simulink model "impulse_ex_3"  (R2024a)
settings: Solver=VariableStepAuto  StartTime=0.0  StopTime=10  RelTol=1e-6  AbsTol=1e-6
values from neighbouring files (symbols this model uses):
  a = 0.001    [impulseDD.sldd]
undefined symbols (not defined in the file or in its folder): sys
libraries: simulink x1
settings Model: DataDictionary=impulseDD.sldd  Creator=grouleau  LastModifiedBy=grouleau

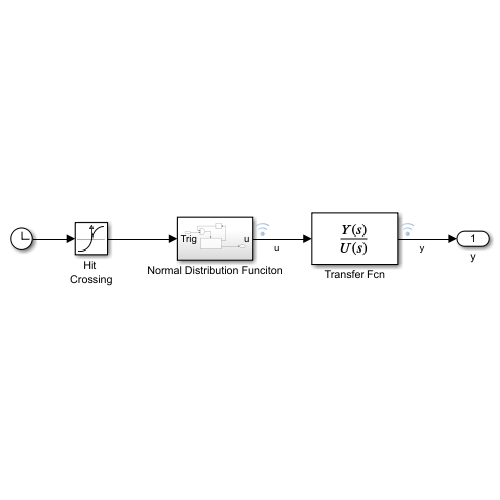
[thumbnail: Simulink's stored preview of the top-level diagram]
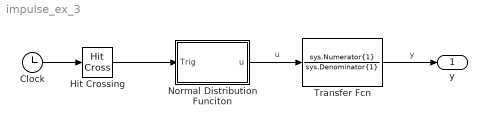
== system impulse_ex_3 ==
  Clock : Clock
  Hit Crossing : HitCross  HitCrossingOffset=1.23456  HitCrossingDirection=rising
  Normal Distribution Funciton : Subsystem
  Transfer Fcn : TransferFcn  Numerator=sys.Numerator{1}  Denominator=sys.Denominator{1}
  y : Outport
  wires:
  Transfer Fcn/1 -> y/1  "y"
  Clock/1 -> Hit Crossing/1
  Normal Distribution Funciton/1(u) -> Transfer Fcn/1  "u"
  Hit Crossing/1 -> Normal Distribution Funciton/1(Trig)

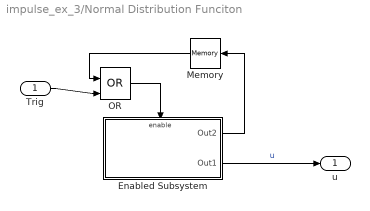
== system impulse_ex_3/Normal Distribution Funciton ==
  Trig : Inport
  Enabled Subsystem : Subsystem  TreatAsAtomicUnit=on
  Memory : Memory
  OR : Logic  Operator=OR  IconShape=distinctive  AllPortsSameDT=off  OutDataTypeStr=boolean
  u : Outport
  wires:
  Enabled Subsystem/2(Out1) -> u/1  "u"
  Enabled Subsystem/1(Out2) -> Memory/1
  OR/1 -> Enabled Subsystem/Enable
  Trig/1 -> OR/2
  Memory/1 -> OR/1

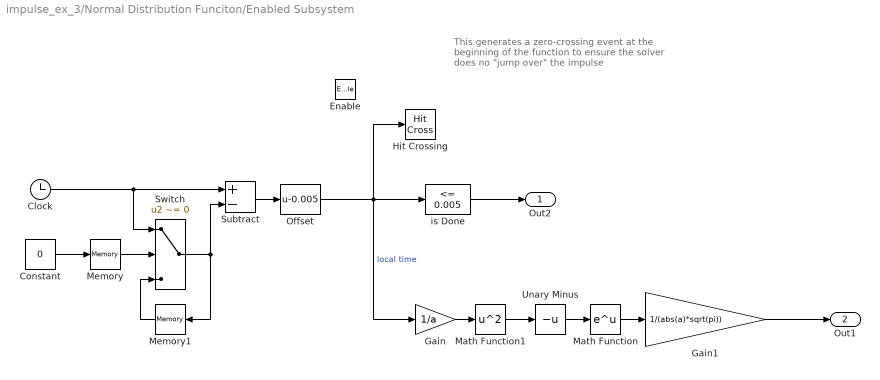
== system impulse_ex_3/Normal Distribution Funciton/Enabled Subsystem ==
  note: This generates a zero-crossing event at the beginning of the function to ensure the solver does no "jump over" the impulse
  Enable : EnablePort  StatesWhenEnabling=reset
  Clock : Clock
  Constant : Constant  Value=0
  Gain : Gain  Gain=1/a
  Gain1 : Gain  Gain=1/(abs(a)*sqrt(pi))
  Hit Crossing : HitCross  HitCrossingOffset=-0.004  ShowOutputPort=off
  Math Function : Math
  Math Function1 : Math  Operator=square
  Memory : Memory  InitialCondition=1
  Memory1 : Memory  InitialCondition=1
  Offset : Bias  Bias=-0.005  SaturateOnIntegerOverflow=off
  Subtract : Sum  Inputs=+-
  Switch : Switch  Criteria=u2 ~= 0  SaturateOnIntegerOverflow=off  InputSameDT=off
  Unary Minus : UnaryMinus
  is Done : simulink/Logic and Bit Operations/Compare To Constant  relop=<=  const=0.005  OutDataTypeStr=boolean
  Out2 : Outport
  Out1 : Outport  Port=2
  wires:
  Clock/1 -> Subtract/1, Switch/1
  Offset/1 -> Gain/1, is Done/1, Hit Crossing/1  "local time"
  Constant/1 -> Memory/1
  Memory/1 -> Switch/2
  Switch/1 -> Subtract/2, Memory1/1
  Memory1/1 -> Switch/3
  Subtract/1 -> Offset/1
  is Done/1 -> Out2/1
  Math Function1/1 -> Unary Minus/1
  Math Function/1 -> Gain1/1
  Gain1/1 -> Out1/1
  Gain/1 -> Math Function1/1
  Unary Minus/1 -> Math Function/1
